simulink model "MultilinkedTilted"  (R2022b)
settings: Solver=FixedStepAuto  StartTime=0.0  StopTime=30  FixedStep=Ts  RelTol=1e-3
InitFcn:
  | % Physical parameters
  | 
  | m = 3.4;
  | m_link = m/4;
  | l = 0.6;
  | beta = 10*2*pi/360;
  | ki = 0.01;
  | 
  | % Control parameters
  | 
  | Kp = diag([2.3, 2.3, 3.6]);
  | Ki = diag([0.02, 0.02, 3.4]);
  | Kd = diag([4, 4, 1.55]);
  | c = 1;
  | 
  | 
  | %% SAMPLING TIME
  | Ts=0.001;
  | 
  | %% PLANNER
  | t_iniz = 0;
  | ttot=20; %duration
  | tdead=10; %dead time to evaluate the steady-state
  | tot_time = ttot + tdead;
  | t1=linspace(0,ttot,round(ttot/Ts));
  | t=linspace(0,ttot+tdead,round(ttot/Ts)+round(tdead/Ts));
  | p= zeros(4,length(t1)); dot_p= zeros(4,length(t1)); ddot_p= zeros(4,length(t1));
  | p_d= zeros(4,length(t)); dot_p_d= zeros(4,length(t)); ddot_p_d= zeros(4,length(t));
  | %Initial and final conditions
  | x0= 0; xf=1; dot_x0= 0; dot_xf=0; ddot_x0=0; ddot_xf=0; dddot_x0 = 0; dddot_xf = 0;
  | y0= 0; yf=1; dot_y0= 0; dot_yf=0; ddot_y0=0; ddot_yf=0; dddot_y0 = 0; dddot_yf = 0;
  | z0= -1; zf=-4; dot_z0= 0; dot_zf=0; ddot_z0=0; ddot_zf=0; dddot_z0 = 0; dddot_zf = 0;
  | psi0 = 0;
  | psif=deg2rad(20); dot_psi0= 0; dot_psif=0; ddot_psi0=0; ddot_psif=0; dddot_psi0 = 0; dddot_psif = 0;
  | p0=[x0,y0,z0,psi0]; dot_p0=[dot_x0,dot_y0,dot_z0,dot_psi0]; ddot_p0=[ddot_x0,ddot_y0,ddot_z0,ddot_psi0]; dddot_p0=[dddot_x0,dddot_y0,dddot_z0,dddot_psi0];
  | pf=[xf,yf,zf,psif]; dot_pf=[dot_xf,dot_yf,dot_zf,dot_psif]; ddot_pf=[ddot_xf,ddot_yf,ddot_zf,ddot_psif]; dddot_pf=[dddot_xf,dddot_yf,dddot_zf,dddot_psif];
  | %5-th order polynomial
  | a0=zeros(1,4); a1=zeros(1,4); a2=zeros(1,4); a3=zeros(1,4); a4=zeros(1,4); a5=zeros(1,4); a6 = zeros(1,4); a7 = zeros(1,4);
  | 
  | for j=1:4
  |     A = [t_iniz^7, t_iniz^6, t_iniz^5, t_iniz^4, t_iniz^3, t_iniz^2, t_iniz, 1;
  |         ttot^7, ttot^6, ttot^5, ttot^4, ttot^3, ttot^2, ttot, 1;
  |         7*t_iniz^6, 6*t_iniz^5, 5*t_iniz^4, 4*t_iniz^3, 3*t_iniz^2, 2*t_iniz, 1, 0;
  |         7*ttot^6, 6*ttot^5, 5*ttot^4, 4*ttot^3, 3*ttot^2, 2*ttot, 1, 0;
  |         42*t_iniz^5, 30*t_iniz^4, 20*t_iniz^3, 12*t_iniz^2, 6*t_iniz, 2, 0, 0;
  |         42*ttot^5, 30*ttot^4, 20*ttot^3, 12*ttot^2, 6*ttot, 2, 0, 0;
  |         210*t_iniz^4, 120*t_iniz^3, 60*t_iniz^2, 24*t_iniz, 6, 0, 0, 0;
  |         210*ttot^4, 120*ttot^3, 60*ttot^2, 24*ttot, 6, 0, 0, 0];
  |     b = [p0(j) pf(j) dot_p0(j) dot_pf(j) ddot_p0(j) ddot_pf(j) dddot_p0(j) dddot_pf(j)]';
  |     a_temp = A\b;
  |     a7(j) = a_temp(1);
  |     a6(j) = a_temp(2);
  |     a5(j) = a_temp(3);
  |     a4(j) = a_temp(4);
  |     a3(j) = a_temp(5);
  |     a2(j) = a_temp(6);
  |     a1(j) = a_temp(7);
  |     a0(j) = a_temp(8);
  | 
  |     %trajectories
  |     p(j,:)=a7(j)*t1.^7 + a6(j)*t1.^6 + a5(j)*t1.^5 +a4(j)*t1.^4 +a3(j)*t1.^3 +a2(j)*t1.^2 +a1(j)*t1 +a0(j);
  |     dot_p(j,:) = 7*a7(j)*t1.^6 + 6*a6(j)*t1.^5 + 5*a5(j)*t1.^4 +4*a4(j)*t1.^3 +3*a3(j)*t1.^2 +2*a2(j)*t1 +a1(j);
  |     ddot_p(j,:) = 42*a7(j)*t1.^5 + 30*a6(j)*t1.^4 + 5*4*a5(j)*t1.^3 +4*3*a4(j)*t1.^2 +3*2*a3(j)*t1 +2*a2(j);
  |     %addition of the stead-state terms
  |     p_d(j,:)=[p(j,:) zeros(1,round(tdead/Ts))+pf(j)];
  |     dot_p_d(j,:)=[dot_p(j,:) zeros(1,round(tdead/Ts))+dot_pf(j)];
  |     ddot_p_d(j,:)=[ddot_p(j,:) zeros(1,round(tdead/Ts))+ddot_pf(j)];
  | end
  | %data for Simulink
  | pos_0 = [x0 y0 z0];
  | lin_vel_0 = [dot_x0 dot_y0 dot_z0];
  | w_bb_0 = [0 0 0];
  | csi_d=p_d(1:3,:); dot_csi_d=dot_p_d(1:3,:); ddot_csi_d=ddot_p_d(1:3,:);
  | psi_d=p_d(4,:); dot_psi_d=dot_p_d(4,:); ddot_psi_d=ddot_p_d(4,:);
values from neighbouring files (symbols this model uses):
  j = j+0.5    (= 0.5)    [PlannerRRT.m]
undefined symbols (not defined in the file or in its folder): DiscIntNeverNeededParam
libraries: simulink x4, robotcorelib x2, uavutilslib x1
settings Model: Creator=Federico  LastModifiedBy=Federico

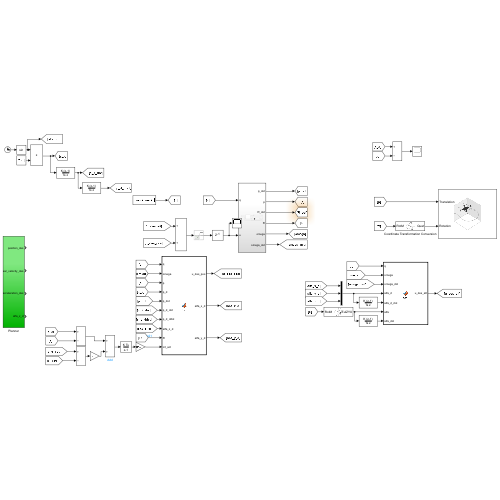
[thumbnail: Simulink's stored preview of the top-level diagram]
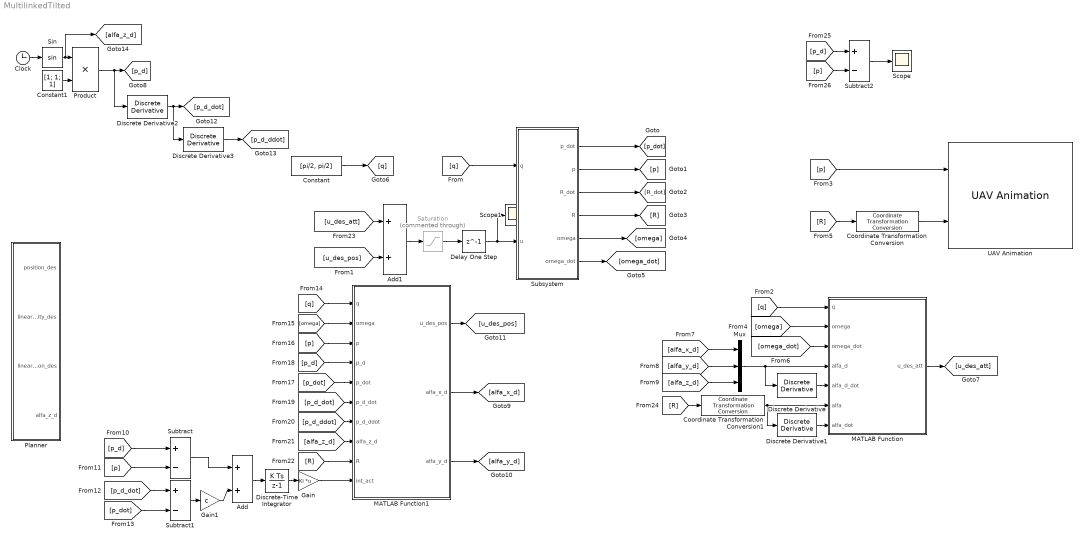
== system MultilinkedTilted ==
  Add : Sum
  Add1 : Sum
  Clock : Clock
  Constant : Constant  Value=[pi/2, pi/2]
  Constant1 : Constant  Value=[1; 1; 1]
  Coordinate Transformation Conversion : robotcorelib/Coordinate Transformation Conversion  InputRepresentation=Rotation Matrix  InputEulerSequence=ZYX  ShowTrVecInputPort=on  OutputRepresentation=Quaternion  OutputEulerSequence=ZYX  ShowTrVecOutputPort=on  SimulateUsing=Interpreted execution
  Coordinate Transformation Conversion1 : robotcorelib/Coordinate Transformation Conversion  InputRepresentation=Rotation Matrix  InputEulerSequence=ZYX  ShowTrVecInputPort=on  OutputRepresentation=Euler Angles  OutputEulerSequence=ZYX  ShowTrVecOutputPort=on  SimulateUsing=Interpreted execution
      settings: LibrarySourceBlock=navlib/Utilities/Coordinate Transformation Conversion
  Delay One Step : Delay  DelayLength=1
  Discrete Derivative{,1..3} (4 alike) : simulink/Discrete/Discrete Derivative  gainval=1.0  ICPrevScaledInput=0.0  OutMin=[]  OutMax=[]  OutDataType=fixdt(1, 16)  OutScaling=2^-10  DoSatur=off
  Discrete-Time Integrator : DiscreteIntegrator  SampleTime=Ts  ICPrevOutput=DiscIntNeverNeededParam  ICPrevScaledInput=DiscIntNeverNeededParam
  Gain : Gain  Gain=Ki  Multiplication=Matrix(K*u)
  Gain1 : Gain  Gain=c
  MATLAB Function : MATLAB Function  TreatAsAtomicUnit=on
  MATLAB Function1 : MATLAB Function  TreatAsAtomicUnit=on
  Mux : Mux  Inputs=3
  Planner : Subsystem
  Product : Product
  Saturation : Saturate  Commented=through  UpperLimit=16  LowerLimit=0
  Scope : Scope
  Scope1 : Scope
  Sin : Trigonometry
  Subsystem : Subsystem
  Subtract : Sum  Inputs=+-
  Subtract1 : Sum  Inputs=+-
  Subtract2 : Sum  Inputs=+-
  UAV Animation : uavutilslib/UAV Animation  UAVType=Multirotor  UAVSize=1  InertialZDirection=Up  SampleTime=0.01
  wires:
  [q] -> Subsystem/1(q)
  Subsystem/1(p_dot) -> [p_dot]
  Subsystem/2(p) -> [p]
  Subsystem/3(R_dot) -> [R_dot]
  Subsystem/4(R) -> [R]
  Subsystem/5(omega) -> [omega]
  Subsystem/6(omega_dot) -> [omega_dot]
  Coordinate Transformation Conversion/1 -> UAV Animation/2
  [p] -> UAV Animation/1
  [R] -> Coordinate Transformation Conversion/1
  Constant/1 -> [q]
  [q] -> MATLAB Function/1(q)
  [omega] -> MATLAB Function/2(omega)
  [omega_dot] -> MATLAB Function/3(omega_dot)
  Mux/1 -> MATLAB Function/4(alfa_d), Discrete Derivative/1
  Discrete Derivative/1 -> MATLAB Function/5(alfa_d_dot)
  MATLAB Function/1(u_des_att) -> [u_des_att]
  [alfa_x_d] -> Mux/1
  [alfa_y_d] -> Mux/2
  [alfa_z_d] -> Mux/3
  Discrete-Time Integrator/1 -> Gain/1
  Gain/1 -> MATLAB Function1/10(int_act)
  Add/1 -> Discrete-Time Integrator/1
  Subtract/1 -> Add/1
  Subtract1/1 -> Gain1/1
  Gain1/1 -> Add/2
  [p_d] -> Subtract/1
  [p] -> Subtract/2
  [p_d_dot] -> Subtract1/1
  [p_dot] -> Subtract1/2
  [q] -> MATLAB Function1/1(q)
  [omega] -> MATLAB Function1/2(omega)
  [p] -> MATLAB Function1/3(p)
  [p_d] -> MATLAB Function1/4(p_d)
  [p_dot] -> MATLAB Function1/5(p_dot)
  [p_d_dot] -> MATLAB Function1/6(p_d_dot)
  [p_d_ddot] -> MATLAB Function1/7(p_d_ddot)
  [alfa_z_d] -> MATLAB Function1/8(alfa_z_d)
  [R] -> MATLAB Function1/9(R)
  MATLAB Function1/2(alfa_x_d) -> [alfa_x_d]
  MATLAB Function1/3(alfa_y_d) -> [alfa_y_d]
  MATLAB Function1/1(u_des_pos) -> [u_des_pos]
  Saturation/1 -> Delay One Step/1
  Add1/1 -> Saturation/1
  [u_des_pos] -> Add1/2
  [u_des_att] -> Add1/1
  Coordinate Transformation Conversion1/1 -> MATLAB Function/6(alfa), Discrete Derivative1/1
  [R] -> Coordinate Transformation Conversion1/1
  Discrete Derivative1/1 -> MATLAB Function/7(alfa_dot)
  Delay One Step/1 -> Scope1/1, Subsystem/2(u)
  [p_d] -> Subtract2/1
  [p] -> Subtract2/2
  Subtract2/1 -> Scope/1
  Clock/1 -> Sin/1
  Sin/1 -> [alfa_z_d], Product/1
  Constant1/1 -> Product/2
  Product/1 -> Discrete Derivative2/1, [p_d]
  Discrete Derivative2/1 -> Discrete Derivative3/1, [p_d_dot]
  Discrete Derivative3/1 -> [p_d_ddot]

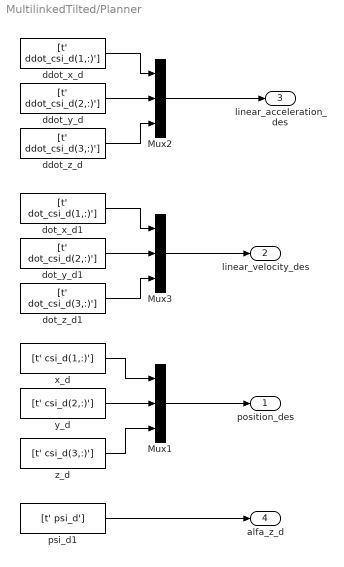
== system MultilinkedTilted/Planner ==
  Mux1 : Mux  Inputs=3
  Mux2 : Mux  Inputs=3
  Mux3 : Mux  Inputs=3
  ddot_x_d : FromWorkspace  VariableName=[t' ddot_csi_d(1,:)']  SampleTime=Ts
  ddot_y_d : FromWorkspace  VariableName=[t' ddot_csi_d(2,:)']  SampleTime=Ts
  ddot_z_d : FromWorkspace  VariableName=[t' ddot_csi_d(3,:)']  SampleTime=Ts
  dot_x_d1 : FromWorkspace  VariableName=[t' dot_csi_d(1,:)']  SampleTime=Ts
  dot_y_d1 : FromWorkspace  VariableName=[t' dot_csi_d(2,:)']  SampleTime=Ts
  dot_z_d1 : FromWorkspace  VariableName=[t' dot_csi_d(3,:)']  SampleTime=Ts
  psi_d1 : FromWorkspace  VariableName=[t' psi_d']  SampleTime=Ts
  x_d : FromWorkspace  VariableName=[t' csi_d(1,:)']  SampleTime=Ts
  y_d : FromWorkspace  VariableName=[t' csi_d(2,:)']  SampleTime=Ts
  z_d : FromWorkspace  VariableName=[t' csi_d(3,:)']  SampleTime=Ts
  position_des : Outport
  linear_velocity_des : Outport  Port=2
  linear_acceleration_des : Outport  Port=3
  alfa_z_d : Outport  Port=4
  wires:
  y_d/1 -> Mux1/2
  z_d/1 -> Mux1/3
  x_d/1 -> Mux1/1
  ddot_y_d/1 -> Mux2/2
  ddot_z_d/1 -> Mux2/3
  ddot_x_d/1 -> Mux2/1
  Mux2/1 -> linear_acceleration_des/1
  Mux1/1 -> position_des/1
  dot_y_d1/1 -> Mux3/2
  dot_z_d1/1 -> Mux3/3
  dot_x_d1/1 -> Mux3/1
  Mux3/1 -> linear_velocity_des/1
  psi_d1/1 -> alfa_z_d/1

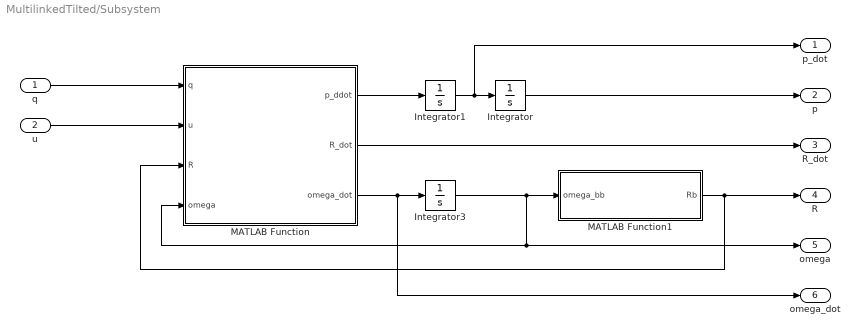
== system MultilinkedTilted/Subsystem ==
  q : Inport
  u : Inport  Port=2
  Integrator : Integrator  InitialCondition=[0 0 1]*0
  Integrator1 : Integrator
  Integrator3 : Integrator
  MATLAB Function : MATLAB Function  TreatAsAtomicUnit=on
  MATLAB Function1 : MATLAB Function  TreatAsAtomicUnit=on
  p_dot : Outport
  p : Outport  Port=2
  R_dot : Outport  Port=3
  R : Outport  Port=4
  omega : Outport  Port=5
  omega_dot : Outport  Port=6
  wires:
  MATLAB Function1/1(Rb) -> MATLAB Function/3(R), R/1
  MATLAB Function/2(R_dot) -> R_dot/1
  MATLAB Function/1(p_ddot) -> Integrator1/1
  Integrator3/1 -> MATLAB Function/4(omega), omega/1, MATLAB Function1/1(omega_bb)
  Integrator1/1 -> p_dot/1, Integrator/1
  MATLAB Function/3(omega_dot) -> omega_dot/1, Integrator3/1
  Integrator/1 -> p/1
  u/1 -> MATLAB Function/2(u)
  q/1 -> MATLAB Function/1(q)

== matlab function MultilinkedTilted/Subsystem/MATLAB Function1 ==
  data: omega_bb input; Rb output
function Rb = fcn(omega_bb)

    Rb = expm(skew(omega_bb));

end

function S = skew(v)
    if(numel(v)~= 1)
        S= [0 -v(3) v(2); 
            v(3) 0 -v(1);
            -v(2) v(1) 0];
    else
        S= zeros(3);
    end
end

== matlab function MultilinkedTilted/Subsystem/MATLAB Function ==
  data: q input size=2; u input; p_ddot output size=3; R_dot output size=[3,3]; R input size=[3,3]; omega input size=3; omega_dot output size=3; m parameter; m_link parameter; l parameter; beta parameter; ki parameter
% UAV model
function [p_ddot, R_dot, omega_dot] = fcn(q, u, R, omega, m, m_link, l, beta, ki)
    
    g = [0; 0; 9.81];
    C1 = [l/2; 0; 0];
    C2 = [l+l/2*cos(q(1)); l/2*sin(q(1)); 0];
    C3 = [l+l*cos(q(1))+l/2*cos(q(1)+pi/2); l*sin(q(1))+l/2*sin(q(1)+pi/2); 0];
    C4 = [l+l*cos(q(1))+l*cos(q(1)+pi/2)+l/2*cos(q(1)+q(2)+pi/2); l*sin(q(1))+l*sin(q(1)+pi/2)+l/2*sin(q(1)+q(2)+pi/2); 0];
    C = (C1+C2+C3+C4)/4;
    r1 = C1-C;
    r2 = C2-C;
    r3 = C3-C;
    r4 = C4-C;
    I_link1 = [0 0 0;
            0 1/12*m_link*l^2 0;
            0 0 1/12*m_link*l^2];
    I_link2 = [cos(q(1)) -sin(q(1)) 0;
        sin(q(1)) cos(q(1)) 0;
        0 0 1]*I_link1*[cos(q(1)) -sin(q(1)) 0;
        sin(q(1)) cos(q(1)) 0;
        0 0 1]';
    I_link3 = [cos(q(1)+pi/2) -sin(q(1)+pi/2) 0;
        sin(q(1)+pi/2) cos(q(1)+pi/2) 0;
        0 0 1]*I_link1*[cos(q(1)+pi/2) -sin(q(1)+pi/2) 0;
        sin(q(1)+pi/2) cos(q(1)+pi/2) 0;
        0 0 1]';
    I_link4 = [cos(q(1)+pi/2+q(2)) -sin(q(1)+pi/2+q(2)) 0;
        sin(q(1)+pi/2+q(2)) cos(q(1)+pi/2+q(2)) 0;
        0 0 1]*I_link1*[cos(q(1)+pi/2+q(2)) -sin(q(1)+pi/2+q(2)) 0;
        sin(q(1)+pi/2+q(2)) cos(q(1)+pi/2+q(2)) 0;
        0 0 1]';
    I = I_link1+I_link2+I_link3+I_link4+m_link*(r1'*r1*eye(3)-r1*r1'+r2'*r2*eye(3)-r2*r2'+r3'*r3*eye(3)-r3*r3'+r4'*r4*eye(3)-r4*r4');

    R_F1C = [cos(-beta) 0 sin(-beta);
        0 1 0;
        -sin(-beta) 0 cos(-beta)];
    
    R_F2C = [cos(q(1)) -sin(q(1)) 0;
        sin(q(1)) cos(q(1)) 0;
        0 0 1]*[cos(beta) 0 sin(beta);
        0 1 0;
        -sin(beta) 0 cos(beta)];
    
    R_F3C = [cos(q(1)+pi/2) -sin(q(1)+pi/2) 0;
        sin(q(1)+pi/2) cos(q(1)+pi/2) 0;
        0 0 1]*[cos(-beta) 0 sin(-beta);
        0 1 0;
        -sin(-beta) 0 cos(-beta)];
    
    R_F4C = [cos(q(1)+pi/2+q(2)) -sin(q(1)+pi/2+q(2)) 0;
        sin(q(1)+pi/2+q(2)) cos(q(1)+pi/2+q(2)) 0;
        0 0 1]*[cos(beta) 0 sin(beta);
        0 1 0;
        -sin(beta) 0 cos(beta)];
    
    Qp_tran = [R_F1C*[0; 0; 1], R_F2C*[0; 0; 1], R_F3C*[0; 0; 1], R_F4C*[0; 0; 1]];
    
    Qp_rot = [(skew(C1-C)+ki*eye(3))*R_F1C*[0; 0; 1], (skew(C2-C)+ki*eye(3))*R_F2C*[0; 0; 1], (skew(C3-C)+ki*eye(3))*R_F3C*[0; 0; 1], (skew(C4-C)+ki*eye(3))*R_F4C*[0; 0; 1]];
    
    up = ([Qp_tran(3,:); Qp_rot])\[1; 0; 0; 0];
    us = m*9.81/norm(Qp_tran*up)*up;
    fs = Qp_tran*us;
    alfa_x = atan2(fs(2), fs(3));
    alfa_y = atan2(-fs(1), sqrt(fs(2)^2+fs(3)^2));
    R_C_CoG = [cos(alfa_y) 0 sin(alfa_y);
        0 1 0;
        -sin(alfa_y) 0 cos(alfa_y)]*[1 0 0;
        0 cos(alfa_x) -sin(alfa_x);
        0 sin(alfa_x) cos(alfa_x)];
    Q_tran = R_C_CoG*Qp_tran;
    Q_rot = R_C_CoG*Qp_rot;

    % u = Q_tran\R'*u;

    p_ddot = 1/m*(R*Q_tran*u)-g;
    omega_dot = I\(-skew(omega)*I*omega+Q_rot*u);
    R_dot = R*skew(omega);

end

function S = skew(v)
    if(numel(v)~= 1)
        S= [0 -v(3) v(2); 
            v(3) 0 -v(1);
            -v(2) v(1) 0];
    else
        S= zeros(3);
    end
end

== matlab function MultilinkedTilted/MATLAB Function ==
  data: q input; u_des_att output size=[4, 1]; m_link parameter; l parameter; omega input; omega_dot input; alfa_d input; alfa_d_dot input; alfa input; alfa_dot input; beta parameter; ki parameter; m parameter
function u_des_att = fcn(q, m_link, l, omega, omega_dot, alfa_d, alfa_d_dot, alfa, alfa_dot, beta, ki, m)

    g = [0; 0; 9.81];
    C1 = [l/2; 0; 0];
    C2 = [l+l/2*cos(q(1)); l/2*sin(q(1)); 0];
    C3 = [l+l*cos(q(1))+l/2*cos(q(1)+pi/2); l*sin(q(1))+l/2*sin(q(1)+pi/2); 0];
    C4 = [l+l*cos(q(1))+l*cos(q(1)+pi/2)+l/2*cos(q(1)+q(2)+pi/2); l*sin(q(1))+l*sin(q(1)+pi/2)+l/2*sin(q(1)+q(2)+pi/2); 0];
    C = (C1+C2+C3+C4)/4;
    r1 = C1-C;
    r2 = C2-C;
    r3 = C3-C;
    r4 = C4-C;
    I_link1 = [0 0 0;
            0 1/12*m_link*l^2 0;
            0 0 1/12*m_link*l^2];
    I_link2 = [cos(q(1)) -sin(q(1)) 0;
        sin(q(1)) cos(q(1)) 0;
        0 0 1]*I_link1*[cos(q(1)) -sin(q(1)) 0;
        sin(q(1)) cos(q(1)) 0;
        0 0 1]';
    I_link3 = [cos(q(1)+pi/2) -sin(q(1)+pi/2) 0;
        sin(q(1)+pi/2) cos(q(1)+pi/2) 0;
        0 0 1]*I_link1*[cos(q(1)+pi/2) -sin(q(1)+pi/2) 0;
        sin(q(1)+pi/2) cos(q(1)+pi/2) 0;
        0 0 1]';
    I_link4 = [cos(q(1)+pi/2+q(2)) -sin(q(1)+pi/2+q(2)) 0;
        sin(q(1)+pi/2+q(2)) cos(q(1)+pi/2+q(2)) 0;
        0 0 1]*I_link1*[cos(q(1)+pi/2+q(2)) -sin(q(1)+pi/2+q(2)) 0;
        sin(q(1)+pi/2+q(2)) cos(q(1)+pi/2+q(2)) 0;
        0 0 1]';
    I = I_link1+I_link2+I_link3+I_link4+m_link*(r1'*r1*eye(3)-r1*r1'+r2'*r2*eye(3)-r2*r2'+r3'*r3*eye(3)-r3*r3'+r4'*r4*eye(3)-r4*r4');

    R_F1C = [cos(-beta) 0 sin(-beta);
        0 1 0;
        -sin(-beta) 0 cos(-beta)];
    
    R_F2C = [cos(q(1)) -sin(q(1)) 0;
        sin(q(1)) cos(q(1)) 0;
        0 0 1]*[cos(beta) 0 sin(beta);
        0 1 0;
        -sin(beta) 0 cos(beta)];
    
    R_F3C = [cos(q(1)+pi/2) -sin(q(1)+pi/2) 0;
        sin(q(1)+pi/2) cos(q(1)+pi/2) 0;
        0 0 1]*[cos(-beta) 0 sin(-beta);
        0 1 0;
        -sin(-beta) 0 cos(-beta)];
    
    R_F4C = [cos(q(1)+pi/2+q(2)) -sin(q(1)+pi/2+q(2)) 0;
        sin(q(1)+pi/2+q(2)) cos(q(1)+pi/2+q(2)) 0;
        0 0 1]*[cos(beta) 0 sin(beta);
        0 1 0;
        -sin(beta) 0 cos(beta)];
    
    Qp_tran = [R_F1C*[0; 0; 1], R_F2C*[0; 0; 1], R_F3C*[0; 0; 1], R_F4C*[0; 0; 1]];
    
    Qp_rot = [(skew(C1-C)+ki*eye(3))*R_F1C*[0; 0; 1], (skew(C2-C)+ki*eye(3))*R_F2C*[0; 0; 1], (skew(C3-C)+ki*eye(3))*R_F3C*[0; 0; 1], (skew(C4-C)+ki*eye(3))*R_F4C*[0; 0; 1]];
    
    up = ([Qp_tran(3,:); Qp_rot])\[1; 0; 0; 0];
    us = m*9.81/norm(Qp_tran*up)*up;
    fs = Qp_tran*us;
    alfa_x = atan2(fs(2), fs(3));
    alfa_y = atan2(-fs(1), sqrt(fs(2)^2+fs(3)^2));
    R_C_CoG = [cos(alfa_y) 0 sin(alfa_y);
        0 1 0;
        -sin(alfa_y) 0 cos(alfa_y)]*[1 0 0;
        0 cos(alfa_x) -sin(alfa_x);
        0 sin(alfa_x) cos(alfa_x)];
    Q_tran = R_C_CoG*Qp_tran;
    Q_rot = R_C_CoG*Qp_rot;

    M = diag([1100, 80, 1100, 800, 10, 50, 10, 10, 0.5]);
    W1 = eye(4);
    W2 = eye(3)*100;
    
    N = W1+Q_tran'*W2*Q_tran;

    A = [0 1 0 0 0 0;
        0 0 0 0 0 0;
        0 0 0 1 0 0;
        0 0 0 0 0 0;
        0 0 0 0 0 1;
        0 0 0 0 0 0];

    B_temp = I\Q_rot;
    B = [0 0 0 0;
        B_temp(1, :);
        0 0 0 0;
        B_temp(2, :);
        0 0 0 0;
        B_temp(3, :)];

    C = [1 0 0 0 0 0;
        0 0 1 0 0 0;
        0 0 0 0 1 0];

    D = [0 0 0;
        1 0 0;
        0 0 0;
        0 1 0;
        0 0 0;
        0 0 1];

    A_bar = [A zeros(6, 3);
        C zeros(3, 3)];

    B_bar = [-B;
        zeros(3, 4)];

    D_bar = [-D;
        zeros(3, 3)];

    Kx = zeros(4, 9) + 1;

    coder.extrinsic('icare');

    [S_care, Kx, L_care] = icare(A_bar, B_bar, M, N);

    x_bar = [alfa_d(1)-alfa(1); alfa_d_dot(1)-alfa_dot(1); alfa_d(2)-alfa(2); alfa_d_dot(1)-alfa_dot(1); alfa_d(3)-alfa(3); alfa_d_dot(1)-alfa_dot(1)];
    x_bar = [x_bar; C*x_bar];

    u_des_att = -Kx*x_bar+Q_rot'*inv(Q_rot*Q_rot')*skew(omega)*I*omega;

end

function S = skew(v)
    if(numel(v)~= 1)
        S= [0 -v(3) v(2); 
            v(3) 0 -v(1);
            -v(2) v(1) 0];
    else
        S= zeros(3);
    end
end

== matlab function MultilinkedTilted/MATLAB Function1 ==
  data: q input; u_des_pos output size=[4, 1]; m_link parameter; l parameter; omega input; p input; p_d input; p_dot input; p_d_dot input; p_d_ddot input; alfa_z_d input; R input; int_act input; beta parameter; ki parameter; m parameter; alfa_x_d output; alfa_y_d output; Kp parameter; Ki parameter; Kd parameter
function [u_des_pos, alfa_x_d, alfa_y_d] = fcn(q, m_link, l, omega, p, p_d, p_dot, p_d_dot, p_d_ddot, alfa_z_d, R, int_act, beta, ki, m, Kp, Ki, Kd)

    g = [0; 0; 9.81];
    C1 = [l/2; 0; 0];
    C2 = [l+l/2*cos(q(1)); l/2*sin(q(1)); 0];
    C3 = [l+l*cos(q(1))+l/2*cos(q(1)+pi/2); l*sin(q(1))+l/2*sin(q(1)+pi/2); 0];
    C4 = [l+l*cos(q(1))+l*cos(q(1)+pi/2)+l/2*cos(q(1)+q(2)+pi/2); l*sin(q(1))+l*sin(q(1)+pi/2)+l/2*sin(q(1)+q(2)+pi/2); 0];
    C = (C1+C2+C3+C4)/4;
    r1 = C1-C;
    r2 = C2-C;
    r3 = C3-C;
    r4 = C4-C;
    I_link1 = [0 0 0;
            0 1/12*m_link*l^2 0;
            0 0 1/12*m_link*l^2];
    I_link2 = [cos(q(1)) -sin(q(1)) 0;
        sin(q(1)) cos(q(1)) 0;
        0 0 1]*I_link1*[cos(q(1)) -sin(q(1)) 0;
        sin(q(1)) cos(q(1)) 0;
        0 0 1]';
    I_link3 = [cos(q(1)+pi/2) -sin(q(1)+pi/2) 0;
        sin(q(1)+pi/2) cos(q(1)+pi/2) 0;
        0 0 1]*I_link1*[cos(q(1)+pi/2) -sin(q(1)+pi/2) 0;
        sin(q(1)+pi/2) cos(q(1)+pi/2) 0;
        0 0 1]';
    I_link4 = [cos(q(1)+pi/2+q(2)) -sin(q(1)+pi/2+q(2)) 0;
        sin(q(1)+pi/2+q(2)) cos(q(1)+pi/2+q(2)) 0;
        0 0 1]*I_link1*[cos(q(1)+pi/2+q(2)) -sin(q(1)+pi/2+q(2)) 0;
        sin(q(1)+pi/2+q(2)) cos(q(1)+pi/2+q(2)) 0;
        0 0 1]';
    I = I_link1+I_link2+I_link3+I_link4+m_link*(r1'*r1*eye(3)-r1*r1'+r2'*r2*eye(3)-r2*r2'+r3'*r3*eye(3)-r3*r3'+r4'*r4*eye(3)-r4*r4');

    R_F1C = [cos(-beta) 0 sin(-beta);
        0 1 0;
        -sin(-beta) 0 cos(-beta)];
    
    R_F2C = [cos(q(1)) -sin(q(1)) 0;
        sin(q(1)) cos(q(1)) 0;
        0 0 1]*[cos(beta) 0 sin(beta);
        0 1 0;
        -sin(beta) 0 cos(beta)];
    
    R_F3C = [cos(q(1)+pi/2) -sin(q(1)+pi/2) 0;
        sin(q(1)+pi/2) cos(q(1)+pi/2) 0;
        0 0 1]*[cos(-beta) 0 sin(-beta);
        0 1 0;
        -sin(-beta) 0 cos(-beta)];
    
    R_F4C = [cos(q(1)+pi/2+q(2)) -sin(q(1)+pi/2+q(2)) 0;
        sin(q(1)+pi/2+q(2)) cos(q(1)+pi/2+q(2)) 0;
        0 0 1]*[cos(beta) 0 sin(beta);
        0 1 0;
        -sin(beta) 0 cos(beta)];
    
    Qp_tran = [R_F1C*[0; 0; 1], R_F2C*[0; 0; 1], R_F3C*[0; 0; 1], R_F4C*[0; 0; 1]];
    
    Qp_rot = [(skew(C1-C)+ki*eye(3))*R_F1C*[0; 0; 1], (skew(C2-C)+ki*eye(3))*R_F2C*[0; 0; 1], (skew(C3-C)+ki*eye(3))*R_F3C*[0; 0; 1], (skew(C4-C)+ki*eye(3))*R_F4C*[0; 0; 1]];
    
    up = ([Qp_tran(3,:); Qp_rot])\[1; 0; 0; 0];
    us = m*9.81/norm(Qp_tran*up)*up;
    fs = Qp_tran*us;
    alfa_x = atan2(fs(2), fs(3));
    alfa_y = atan2(-fs(1), sqrt(fs(2)^2+fs(3)^2));
    R_C_CoG = [cos(alfa_y) 0 sin(alfa_y);
        0 1 0;
        -sin(alfa_y) 0 cos(alfa_y)]*[1 0 0;
        0 cos(alfa_x) -sin(alfa_x);
        0 sin(alfa_x) cos(alfa_x)];
    Q_tran = R_C_CoG*Qp_tran;
    Q_rot = R_C_CoG*Qp_rot;

    er = p_d-p;
    er_dot = p_d_dot-p_dot;

    f_des = m*(Kp*er+int_act+Kd*er_dot+p_d_ddot)-R_C_CoG*Q_tran*Q_rot'*inv(Q_rot*Q_rot')*skew(omega)*I*omega;
    f_bar = [cos(alfa_z_d) -sin(alfa_z_d) 0;
             sin(alfa_z_d) cos(alfa_z_d)  0;
             0             0              1]\f_des;
    alfa_x_d = atan2(-f_bar(2), sqrt(f_bar(1)^2+f_bar(3)^2));
    alfa_y_d = atan2(f_bar(1), f_bar(3));
    f_des_T = (R*[0; 0; 1])'*f_des;

    u_des_pos = us/(m*9.81)*f_des_T;

end

function S = skew(v)
    if(numel(v)~= 1)
        S= [0 -v(3) v(2); 
            v(3) 0 -v(1);
            -v(2) v(1) 0];
    else
        S= zeros(3);
    end
end
